simulink model "VerificationSSMRec2016A"  (R2016a)
settings: Solver=ode4  StartTime=0.0  StopTime=Tfinal  FixedStep=Ts  RelTol=1e-3
values from neighbouring files (symbols this model uses):
  Cdc = 15e-6    (= 1.5e-05)    [sim_parameters.m]    (also in stateSpaceEnes.m)
  Cdcrec = 1e-3    (= 0.001)    [sim_parameters.m]    (also in stateSpaceEnes.m)
  delta = 0    [sim_parameters.m]    (also in stateSpaceEnes.m)
  LA = 15e-3    (= 0.015)    [sim_parameters.m]    (also in stateSpaceEnes.m)
  LB = 15e-3    (= 0.015)    [sim_parameters.m]    (also in stateSpaceEnes.m)
  LC = 15e-3    (= 0.015)    [sim_parameters.m]    (also in stateSpaceEnes.m)
  Lin = 3.4e-5    (= 3.4e-05)    [sim_parameters.m]    (also in stateSpaceEnes.m)
  ma1 = 0.9    [sim_parameters.m]
  phase = 0    [sim_parameters.m]
  RA = 10    [sim_parameters.m]    (also in stateSpaceEnes.m = 10.000001)
  RB = 10    [sim_parameters.m]    (also in stateSpaceEnes.m = 10.000001)
  RC = 10    [sim_parameters.m]    (also in stateSpaceEnes.m = 10.000001)
  Rin = 2    [sim_parameters.m]    (also in stateSpaceEnes.m)
  Ts = 1e-6    (= 1e-06)    [sim_parameters.m]
  Vin = 130    [sim_parameters.m]
  wout = 2*pi*fout    (= 314.159265359)    [sim_parameters.m]
undefined symbols (not defined in the file or in its folder): Lload, Rload
libraries: powerlib x25, powerlib_meascontrol x10
settings Model: SimulationMode=accelerator  Creator=ugurm  LastModifiedBy=enes_
settings DataIOCC: LimitDataPoints=on  SaveFormat=Array
settings DebuggingCC: UnderspecifiedInitializationDetection=Classic  MergeDetectMultiDrivingBlocksExec=none  SolverPrmCheckMsg=warning  StateNameClashWarn=warning
settings HardwareCC: ProdBitPerPointer=32  ProdLargestAtomicFloat=None  ProdIntDivRoundTo=Undefined  ProdEndianess=Unspecified  ProdWordSize=32  ProdHWDeviceType=32-bit Generic
settings ModelReferenceCC: PropagateSignalLabelsOutOfModel=off
settings SimscapeCC: SimscapeNormalizeSystem=off

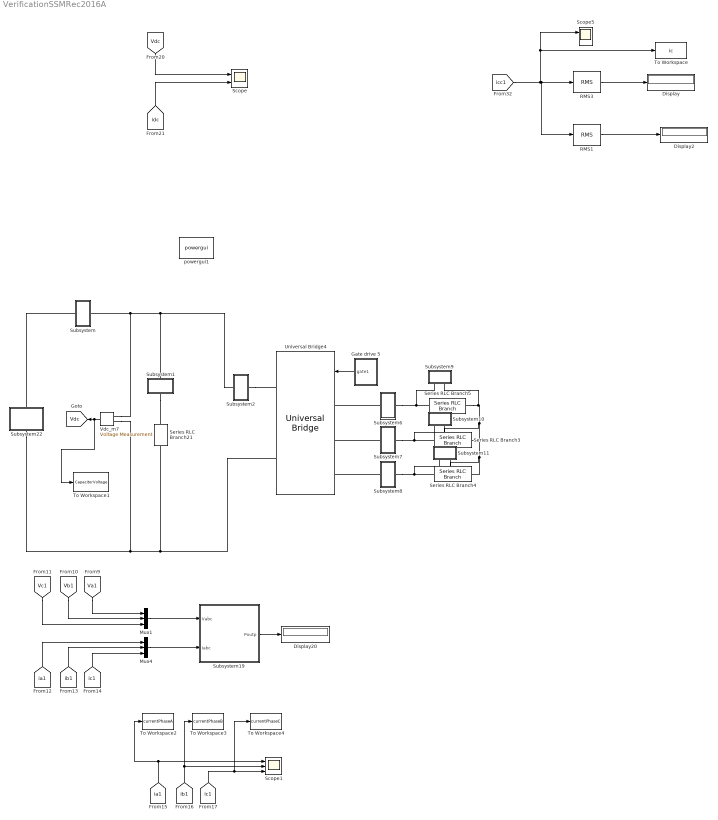
== system VerificationSSMRec2016A ==
  Display : Display
  Display2 : Display
  Display20 : Display
  Gate drive 5 : Subsystem
  Mux1 : Mux  Inputs=3
  Mux4 : Mux  Inputs=3
  RMS1 : powerlib_meascontrol/Measurements/RMS  TrueRMS=on  Freq=fsw  RMSInit=0  Ts=0
  RMS3 : powerlib_meascontrol/Measurements/RMS  TrueRMS=on  Freq=fout  RMSInit=0  Ts=0
  Scope : Scope  NumInputPorts=2
  Scope1 : Scope  NumInputPorts=3
  Scope5 : Scope  NumInputPorts=2
  Series RLC Branch21 : powerlib/Elements/Series RLC Branch  LConnTagsString=__new0  RConnTagsString=__new0  BranchType=C  Resistance=Rload  Inductance=Lload  SetiL0=off  InitialCurrent=0  Capacitance=Cdc  Setx0=off  InitialVoltage=0  Measurements=None
  Series RLC Branch3 : powerlib/Elements/Series RLC Branch  LConnTagsString=__new0  RConnTagsString=__new0  BranchType=RL  Resistance=RB  Inductance=LB  SetiL0=off  InitialCurrent=0  Capacitance=1e-6  Setx0=off  InitialVoltage=0  Measurements=None
  Series RLC Branch4 : powerlib/Elements/Series RLC Branch  LConnTagsString=__new0  RConnTagsString=__new0  BranchType=RL  Resistance=RC  Inductance=LC  SetiL0=off  InitialCurrent=0  Capacitance=1e-6  Setx0=off  InitialVoltage=0  Measurements=None
  Series RLC Branch5 : powerlib/Elements/Series RLC Branch  LConnTagsString=__new0  RConnTagsString=__new0  BranchType=RL  Resistance=RA  Inductance=LA  SetiL0=off  InitialCurrent=0  Capacitance=1e-6  Setx0=off  InitialVoltage=0  Measurements=None
  Subsystem : Subsystem
  Subsystem1 : Subsystem
  Subsystem10 : Subsystem
  Subsystem11 : Subsystem
  Subsystem19 : Subsystem
  Subsystem2 : Subsystem
  Subsystem22 : Subsystem
  Subsystem6 : Subsystem
  Subsystem7 : Subsystem
  Subsystem8 : Subsystem
  Subsystem9 : Subsystem
  To Workspace : ToWorkspace  VariableName=ic  SaveFormat=Timeseries  SampleTime=-1
  To Workspace1 : ToWorkspace  VariableName=CapacitorVoltage  SaveFormat=Timeseries  SampleTime=-1
  To Workspace2 : ToWorkspace  VariableName=currentPhaseA  SaveFormat=Timeseries  SampleTime=-1
  To Workspace3 : ToWorkspace  VariableName=currentPhaseB  SaveFormat=Timeseries  SampleTime=-1
  To Workspace4 : ToWorkspace  VariableName=currentPhaseC  SaveFormat=Timeseries  SampleTime=-1
  Universal Bridge4 : powerlib/Power Electronics/Universal Bridge  Arms=3  SnubberResistance=1e5  SnubberCapacitance=inf  Device=IGBT / Diodes  Ron=1e-6  Lon=0  ForwardVoltages="[  0  0  ]"  ForwardVoltage=0  GTOparameters=[ 10e-6 , 20e-6 ]  IGBTparameters=[0,0]  Measurements=None  Measurements_2=None  converterType=Rectifier
  Vdc_m7 : powerlib/Measurements/Voltage Measurement  PhasorSimulation=off  OutputType=Complex  PSBequivalent=0
  powergui1 : powerlib/powergui  Priority=1  SimulationMode=Discrete  SampleTime=Ts  frequency=60  Iterations=50  frequencyindice=0  Pbase=100e6  ErrMax=1e-4  UnitsV=kV  UnitsW=MW  buscounter=0  FunctionMessages=off  echomessages=off  EnableUseOfTLC=off  CurrentSourceSwitches=off  DisableSnubberDevices=off  DisableRonSwitches=off  DisableVfSwitches=off  DisplayEquations=off  SolverType=Tustin  Interpol=off  ExternalGateDelay=off  methode=off  Ts=0  x0status=blocks  SPID=off  SwTol=0  HookPort=off  RestoreLinks=warning  ResistiveCurrentMeasurement=off  Frange=[0:2:500]  Ylog=off  Xlog=on  ShowGrid=off  save=off  variable=ZData  structure=Vdc  ZoomFFT=off  StartTime=0.04  cycles=5  DisplayStyle=5  fundamental=50  FreqAxis=off  MaxFrequency=30000  frequencyindicesteady=1  RmsSteady=1  display=off
  tag scope: Vdc=global
  wires:
  Vdc_m7/1 -> To Workspace1/1, [Vdc]
  Gate drive 5/1(gate1) -> Universal Bridge4/1
  Subsystem19/1(Poutp) -> Display20/1
  [ic1] -> Mux4/3
  Mux4/1 -> Subsystem19/2(Iabc)
  Mux1/1 -> Subsystem19/1(Vabc)
  [ia1] -> Mux4/1
  [ib1] -> Mux4/2
  [Va1] -> Mux1/1
  [Vb1] -> Mux1/2
  [Vc1] -> Mux1/3
  [ic1] -> To Workspace4/1, Scope1/3
  [ia1] -> Scope1/1, To Workspace2/1
  [Vdc] -> Scope/1
  [idc] -> Scope/2
  RMS3/1 -> Display/1
  [icc1] -> Scope5/1, To Workspace/1, RMS1/1, RMS3/1
  RMS1/1 -> Display2/1
  [ib1] -> To Workspace3/1, Scope1/2
  connections:
  Subsystem1/RConn1 -- Series RLC Branch21/LConn1
  Vdc_m7/LConn1 -- Subsystem1/LConn1 -- Subsystem2/LConn1 -- Subsystem/RConn1
  Vdc_m7/LConn2 -- Series RLC Branch21/RConn1 -- Universal Bridge4/RConn2 -- Subsystem22/LConn1
  Subsystem6/LConn1 -- Universal Bridge4/LConn1
  Subsystem8/LConn1 -- Universal Bridge4/LConn3
  Subsystem7/LConn1 -- Universal Bridge4/LConn2
  Subsystem8/RConn1 -- Subsystem11/LConn1 -- Series RLC Branch4/LConn1
  Subsystem7/RConn1 -- Subsystem10/LConn1 -- Series RLC Branch3/LConn1
  Series RLC Branch5/RConn1 -- Subsystem9/LConn2 -- Subsystem10/LConn2 -- Subsystem11/LConn2 -- Series RLC Branch4/RConn1 -- Series RLC Branch3/RConn1
  Subsystem6/RConn1 -- Subsystem9/LConn1 -- Series RLC Branch5/LConn1
  Subsystem22/RConn1 -- Subsystem/LConn1
  Subsystem2/RConn1 -- Universal Bridge4/RConn1

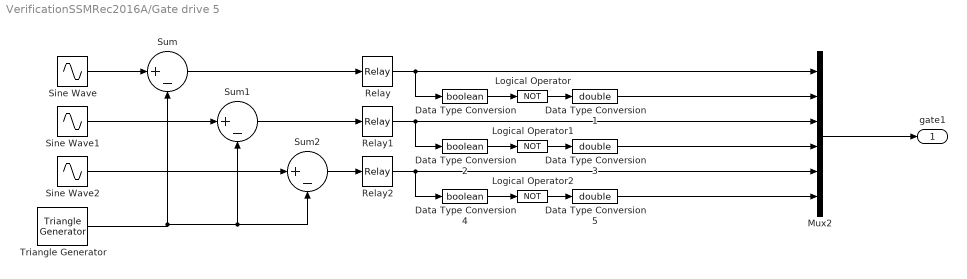
== system VerificationSSMRec2016A/Gate drive 5 ==
  Data Type Conversion : DataTypeConversion  OutDataTypeStr=boolean
  Data Type Conversion1 : DataTypeConversion  OutDataTypeStr=double
  Data Type Conversion2 : DataTypeConversion  OutDataTypeStr=boolean
  Data Type Conversion3 : DataTypeConversion  OutDataTypeStr=double
  Data Type Conversion4 : DataTypeConversion  OutDataTypeStr=boolean
  Data Type Conversion5 : DataTypeConversion  OutDataTypeStr=double
  Logical Operator : Logic  Operator=NOT  AllPortsSameDT=off  OutDataTypeStr=boolean
  Logical Operator1 : Logic  Operator=NOT  AllPortsSameDT=off  OutDataTypeStr=boolean
  Logical Operator2 : Logic  Operator=NOT  AllPortsSameDT=off  OutDataTypeStr=boolean
  Mux2 : Mux  Inputs=6
  Relay : Relay
  Relay1 : Relay
  Relay2 : Relay
  Sine Wave : Sin  Amplitude=ma1  Frequency=wout  Phase=delta  SampleTime=0
  Sine Wave1 : Sin  Amplitude=ma1  Frequency=wout  Phase=-2*pi/3+delta  SampleTime=0
  Sine Wave2 : Sin  Amplitude=ma1  Frequency=wout  Phase=2*pi/3+delta  SampleTime=0
  Sum : Sum  Inputs=|+-
  Sum1 : Sum  Inputs=|+-
  Sum2 : Sum  Inputs=|+-
  Triangle Generator : powerlib_meascontrol/Pulse & Signal Generators/Triangle Generator  Freq=fsw  Phase=phase  Ts=Ts
  gate1 : Outport
  wires:
  Sine Wave/1 -> Sum/1
  Triangle Generator/1 -> Sum1/2, Sum2/2, Sum/2
  Sine Wave1/1 -> Sum1/1
  Sine Wave2/1 -> Sum2/1
  Sum/1 -> Relay/1
  Sum1/1 -> Relay1/1
  Sum2/1 -> Relay2/1
  Data Type Conversion/1 -> Logical Operator/1
  Relay/1 -> Data Type Conversion/1, Mux2/1
  Logical Operator/1 -> Data Type Conversion1/1
  Data Type Conversion1/1 -> Mux2/2
  Data Type Conversion2/1 -> Logical Operator1/1
  Relay1/1 -> Data Type Conversion2/1, Mux2/3
  Logical Operator1/1 -> Data Type Conversion3/1
  Data Type Conversion3/1 -> Mux2/4
  Data Type Conversion4/1 -> Logical Operator2/1
  Relay2/1 -> Data Type Conversion4/1, Mux2/5
  Logical Operator2/1 -> Data Type Conversion5/1
  Data Type Conversion5/1 -> Mux2/6
  Mux2/1 -> gate1/1

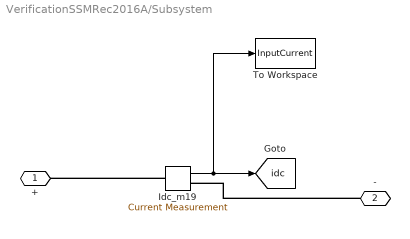
== system VerificationSSMRec2016A/Subsystem ==
  Idc_m19 : powerlib/Measurements/Current Measurement  PhasorSimulation=off  OutputType=Complex  PSBequivalent=0
  To Workspace : ToWorkspace  VariableName=InputCurrent  SaveFormat=Timeseries  SampleTime=-1
  + : PMIOPort  Side=Left
  " -" : PMIOPort  Port=2  Side=Right
  tag scope: idc=global
  wires:
  Idc_m19/1 -> To Workspace/1, [idc]
  connections:
  " -"/RConn1 -- Idc_m19/RConn1
  Idc_m19/LConn1 -- +/RConn1

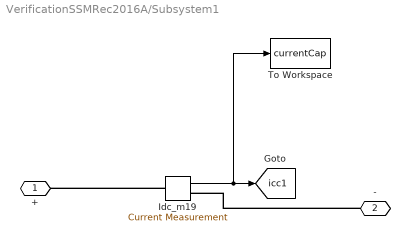
== system VerificationSSMRec2016A/Subsystem1 ==
  Idc_m19 : powerlib/Measurements/Current Measurement  PhasorSimulation=off  OutputType=Complex  PSBequivalent=0
  To Workspace : ToWorkspace  VariableName=currentCap  SaveFormat=Timeseries  SampleTime=-1
  + : PMIOPort  Side=Left
  " -" : PMIOPort  Port=2  Side=Right
  tag scope: icc1=global
  wires:
  Idc_m19/1 -> To Workspace/1, [icc1]
  connections:
  " -"/RConn1 -- Idc_m19/RConn1
  Idc_m19/LConn1 -- +/RConn1

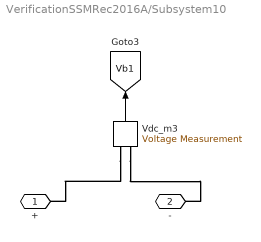
== system VerificationSSMRec2016A/Subsystem10 ==
  Vdc_m3 : powerlib/Measurements/Voltage Measurement  PhasorSimulation=off  OutputType=Complex  PSBequivalent=0
  + : PMIOPort  Side=Left
  - : PMIOPort  Port=2  Side=Left
  tag scope: Vb1=global
  wires:
  Vdc_m3/1 -> [Vb1]
  connections:
  Vdc_m3/LConn1 -- +/RConn1
  Vdc_m3/LConn2 -- -/RConn1

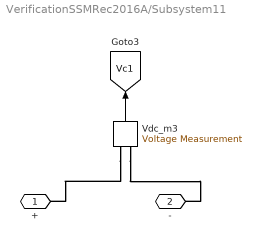
== system VerificationSSMRec2016A/Subsystem11 ==
  Vdc_m3 : powerlib/Measurements/Voltage Measurement  PhasorSimulation=off  OutputType=Complex  PSBequivalent=0
  + : PMIOPort  Side=Left
  - : PMIOPort  Port=2  Side=Left
  tag scope: Vc1=global
  wires:
  Vdc_m3/1 -> [Vc1]
  connections:
  Vdc_m3/LConn1 -- +/RConn1
  Vdc_m3/LConn2 -- -/RConn1

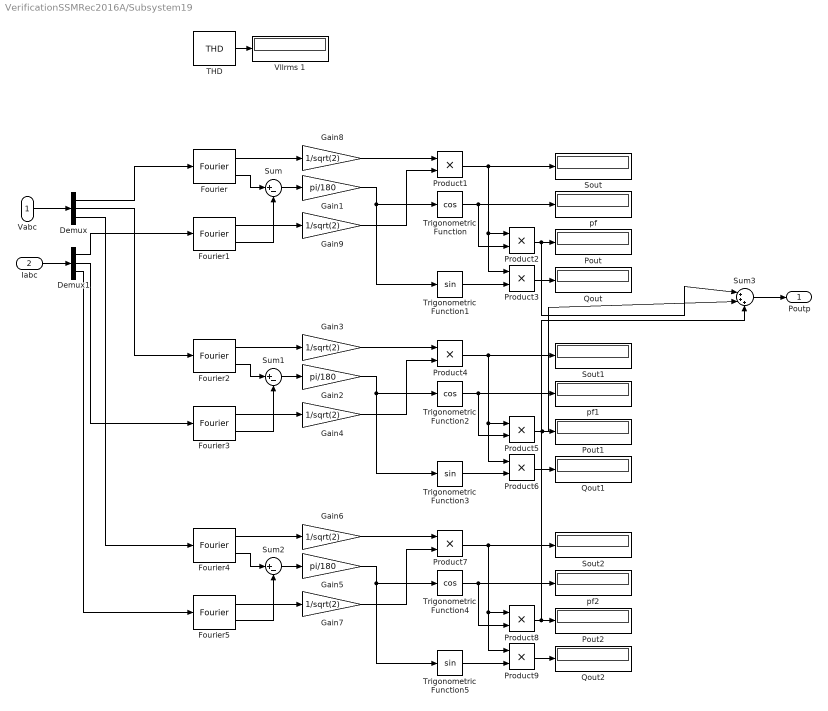
== system VerificationSSMRec2016A/Subsystem19 ==
  Vabc : Inport
  Iabc : Inport  Port=2
  Demux : Demux  Outputs=3
  Demux1 : Demux  Outputs=3
  Fourier{,1..5} (6 alike) : powerlib_meascontrol/Measurements/Fourier  Freq=fout  n=1  InInit=[0, 0]  Ts=Ts
  Gain1 : Gain  Gain=pi/180
  Gain2 : Gain  Gain=pi/180
  Gain{3..4,6..9} (6 alike) : Gain  Gain=1/sqrt(2)
  Gain5 : Gain  Gain=pi/180
  Pout : Display
  Pout1 : Display
  Pout2 : Display
  Product{1..9} (9 alike) : Product
  Qout : Display
  Qout1 : Display
  Qout2 : Display
  Sout : Display
      settings: Format=short_e
  Sout1 : Display
      settings: Format=short_e
  Sout2 : Display
      settings: Format=short_e
  Sum : Sum  Inputs=|+-
  Sum1 : Sum  Inputs=|+-
  Sum2 : Sum  Inputs=|+-
  Sum3 : Sum  Inputs=|+++
  THD : powerlib_meascontrol/Measurements/THD  Freq=fout  Ts=0
  Trigonometric Function : Trigonometry  Operator=cos
  Trigonometric Function1 : Trigonometry
  Trigonometric Function2 : Trigonometry  Operator=cos
  Trigonometric Function3 : Trigonometry
  Trigonometric Function4 : Trigonometry  Operator=cos
  Trigonometric Function5 : Trigonometry
  Vllrms 1 : Display
  pf : Display
  pf1 : Display
  pf2 : Display
  Poutp : Outport
  wires:
  Gain8/1 -> Product1/1
  Gain9/1 -> Product1/2
  Fourier1/1 -> Gain9/1
  Fourier/1 -> Gain8/1
  Product1/1 -> Product3/1, Product2/1, Sout/1
  Sum/1 -> Gain1/1
  Trigonometric Function/1 -> Product2/2, pf/1
  Gain1/1 -> Trigonometric Function1/1, Trigonometric Function/1
  Product2/1 -> Sum3/1, Pout/1
  THD/1 -> Vllrms 1/1
  Vabc/1 -> Demux/1
  Iabc/1 -> Demux1/1
  Fourier/2 -> Sum/1
  Fourier1/2 -> Sum/2
  Trigonometric Function1/1 -> Product3/2
  Product3/1 -> Qout/1
  Gain3/1 -> Product4/1
  Gain4/1 -> Product4/2
  Fourier3/1 -> Gain4/1
  Fourier2/1 -> Gain3/1
  Product4/1 -> Product6/1, Product5/1, Sout1/1
  Sum1/1 -> Gain2/1
  Trigonometric Function2/1 -> Product5/2, pf1/1
  Gain2/1 -> Trigonometric Function3/1, Trigonometric Function2/1
  Product5/1 -> Sum3/2, Pout1/1
  Fourier2/2 -> Sum1/1
  Fourier3/2 -> Sum1/2
  Trigonometric Function3/1 -> Product6/2
  Product6/1 -> Qout1/1
  Gain6/1 -> Product7/1
  Gain7/1 -> Product7/2
  Fourier5/1 -> Gain7/1
  Fourier4/1 -> Gain6/1
  Product7/1 -> Product9/1, Product8/1, Sout2/1
  Sum2/1 -> Gain5/1
  Trigonometric Function4/1 -> Product8/2, pf2/1
  Gain5/1 -> Trigonometric Function5/1, Trigonometric Function4/1
  Fourier4/2 -> Sum2/1
  Fourier5/2 -> Sum2/2
  Trigonometric Function5/1 -> Product9/2
  Product9/1 -> Qout2/1
  Product8/1 -> Sum3/3, Pout2/1
  Sum3/1 -> Poutp/1
  Demux/1 -> Fourier/1
  Demux/2 -> Fourier2/1
  Demux/3 -> Fourier4/1
  Demux1/1 -> Fourier1/1
  Demux1/2 -> Fourier3/1
  Demux1/3 -> Fourier5/1

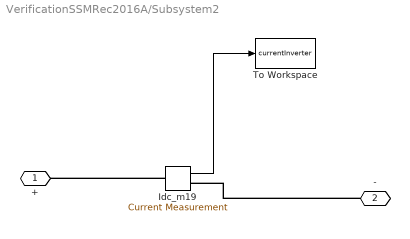
== system VerificationSSMRec2016A/Subsystem2 ==
  Idc_m19 : powerlib/Measurements/Current Measurement  PhasorSimulation=off  OutputType=Complex  PSBequivalent=0
  To Workspace : ToWorkspace  VariableName=currentInverter  SaveFormat=Timeseries  SampleTime=-1
  + : PMIOPort  Side=Left
  " -" : PMIOPort  Port=2  Side=Right
  wires:
  Idc_m19/1 -> To Workspace/1
  connections:
  " -"/RConn1 -- Idc_m19/RConn1
  Idc_m19/LConn1 -- +/RConn1

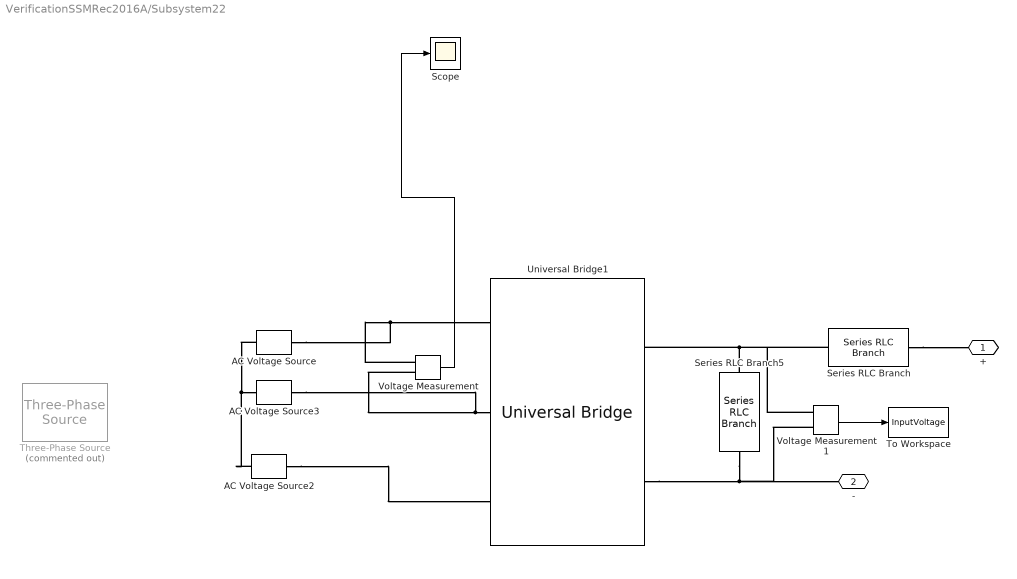
== system VerificationSSMRec2016A/Subsystem22 ==
  AC Voltage Source : powerlib/Electrical Sources/AC Voltage Source  Amplitude=Vin/(sqrt(3))  Phase=0  Frequency=50  SampleTime=0  Measurements=None  BusType=swing  Pref=10e3  Qref=0  Qmin=-inf  Qmax=+inf
  AC Voltage Source2 : powerlib/Electrical Sources/AC Voltage Source  Amplitude=Vin/(sqrt(1)*sqrt(3))  Phase=+120  Frequency=50  SampleTime=0  Measurements=None  BusType=swing  Pref=10e3  Qref=0  Qmin=-inf  Qmax=+inf
  AC Voltage Source3 : powerlib/Electrical Sources/AC Voltage Source  Amplitude=Vin/(sqrt(1)*sqrt(3))  Phase=-120  Frequency=50  SampleTime=0  Measurements=None  BusType=swing  Pref=10e3  Qref=0  Qmin=-inf  Qmax=+inf
  Scope : Scope
  Series RLC Branch : powerlib/Elements/Series RLC Branch  LConnTagsString=__new0  RConnTagsString=__new0  BranchType=RL  Resistance=Rin  Inductance=Lin  SetiL0=off  InitialCurrent=0  Capacitance=1e-6  Setx0=off  InitialVoltage=0  Measurements=None
  Series RLC Branch5 : powerlib/Elements/Series RLC Branch  LConnTagsString=__new0  RConnTagsString=__new0  BranchType=C  Resistance=Rload  Inductance=Lload  SetiL0=off  InitialCurrent=0  Capacitance=Cdcrec  Setx0=on  InitialVoltage=0  Measurements=None
  Three-Phase Source : powerlib/Electrical Sources/Three-Phase Source  Commented=on  InternalConnection=Yg  VoltagePhases=off  Voltage=Vin/sqrt(2)  PhaseAngle=delta  Voltage_phases=[25e3 25e3 25e3]/sqrt(3)  PhaseAngles_phases=[0 -120 +120]  Frequency=50  NonIdealSource=on  SpecifyImpedance=off  Resistance=0.8929  Inductance=16.58e-3  ShortCircuitLevel=100e6  BaseVoltage=25e3  XRratio=7  BusType=swing  Pref=10e3  Qref=0  Prefabc=[10e3, 10e3, 10e3]  Qrefabc=[0, 0, 0]  Qmin=-inf  Qmax=inf
  To Workspace : ToWorkspace  VariableName=InputVoltage  SaveFormat=Timeseries  SampleTime=-1
  Universal Bridge1 : powerlib/Power Electronics/Universal Bridge  Arms=3  SnubberResistance=1e5  SnubberCapacitance=inf  Device=Diodes  Ron=1e-6  Lon=0  ForwardVoltages="[  0  0  ]"  ForwardVoltage=0  GTOparameters=[ 10e-6 , 20e-6 ]  IGBTparameters=[0,0]  Measurements=None  Measurements_2=None  converterType=Rectifier
  Voltage Measurement : powerlib/Measurements/Voltage Measurement  PhasorSimulation=off  OutputType=Complex  PSBequivalent=0
  Voltage Measurement1 : powerlib/Measurements/Voltage Measurement  PhasorSimulation=off  OutputType=Complex  PSBequivalent=0
  + : PMIOPort  Side=Right
  - : PMIOPort  Port=2  Side=Left
  wires:
  Voltage Measurement/1 -> Scope/1
  Voltage Measurement1/1 -> To Workspace/1
  connections:
  Series RLC Branch5/LConn1 -- Voltage Measurement1/LConn1 -- Series RLC Branch/LConn1 -- Universal Bridge1/RConn1
  Universal Bridge1/RConn2 -- Series RLC Branch5/RConn1 -- -/RConn1 -- Voltage Measurement1/LConn2
  Voltage Measurement/LConn2 -- AC Voltage Source3/RConn1 -- Universal Bridge1/LConn2
  Voltage Measurement/LConn1 -- AC Voltage Source/RConn1 -- Universal Bridge1/LConn1
  Series RLC Branch/RConn1 -- +/RConn1
  AC Voltage Source2/RConn1 -- Universal Bridge1/LConn3
  AC Voltage Source/LConn1 -- AC Voltage Source2/LConn1 -- AC Voltage Source3/LConn1

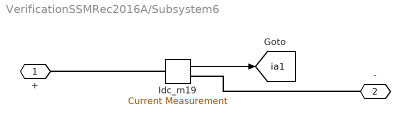
== system VerificationSSMRec2016A/Subsystem6 ==
  Idc_m19 : powerlib/Measurements/Current Measurement  PhasorSimulation=off  OutputType=Complex  PSBequivalent=0
  + : PMIOPort  Side=Left
  " -" : PMIOPort  Port=2  Side=Right
  tag scope: ia1=global
  wires:
  Idc_m19/1 -> [ia1]
  connections:
  " -"/RConn1 -- Idc_m19/RConn1
  Idc_m19/LConn1 -- +/RConn1

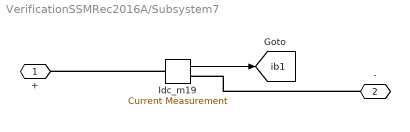
== system VerificationSSMRec2016A/Subsystem7 ==
  Idc_m19 : powerlib/Measurements/Current Measurement  PhasorSimulation=off  OutputType=Complex  PSBequivalent=0
  + : PMIOPort  Side=Left
  " -" : PMIOPort  Port=2  Side=Right
  tag scope: ib1=global
  wires:
  Idc_m19/1 -> [ib1]
  connections:
  " -"/RConn1 -- Idc_m19/RConn1
  Idc_m19/LConn1 -- +/RConn1

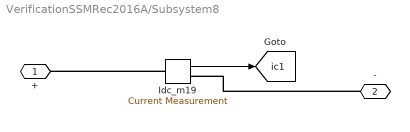
== system VerificationSSMRec2016A/Subsystem8 ==
  Idc_m19 : powerlib/Measurements/Current Measurement  PhasorSimulation=off  OutputType=Complex  PSBequivalent=0
  + : PMIOPort  Side=Left
  " -" : PMIOPort  Port=2  Side=Right
  tag scope: ic1=global
  wires:
  Idc_m19/1 -> [ic1]
  connections:
  " -"/RConn1 -- Idc_m19/RConn1
  Idc_m19/LConn1 -- +/RConn1

== system VerificationSSMRec2016A/Subsystem9 ==
  Vdc_m3 : powerlib/Measurements/Voltage Measurement  PhasorSimulation=off  OutputType=Complex  PSBequivalent=0
  + : PMIOPort  Side=Left
  - : PMIOPort  Port=2  Side=Left
  tag scope: Va1=global
  wires:
  Vdc_m3/1 -> [Va1]
  connections:
  Vdc_m3/LConn1 -- +/RConn1
  Vdc_m3/LConn2 -- -/RConn1
